simulink model "two_tanks_start"  (R2018a)
settings: Solver=ode45  StartTime=0.0  StopTime=250  RelTol=1e-3  EnableMultiTasking=on
PreLoadFcn:
  | rho = 1000;
  | A = 4;
  | g = 9.81;
  | R = 5;
  | W_in = 100;
  | h0 = 0;
  | hmax = 2;
settings Model: Creator=nicholas  LastModifiedBy=bneiswan
settings DataIOCC: LimitDataPoints=on  SaveFormat=Array  SignalLoggingName=sigsOut
settings OptimizationCC: BooleanDataType=off  OptimizeBlockIOStorage=off  BufferReuse=off  GlobalBufferReuse=off  ExpressionFolding=off  ExpressionDepthLimit=2147483647  LocalBlockOutputs=off  InitFltsAndDblsToZero=on  LifeSpan=inf  OptimizeDataStoreBuffers=off  BusAssignmentInplaceUpdate=off
settings DebuggingCC: SaveWithParameterizedLinksMsg=none  UnderspecifiedInitializationDetection=Classic  MergeDetectMultiDrivingBlocksExec=none  CheckExecutionContextPreStartOutputMsg=on  CheckExecutionContextRuntimeOutputMsg=on  SignalResolutionControl=TryResolveAllWithWarning  MultiTaskDSMMsg=warning  MultiTaskCondExecSysMsg=none  ParameterPrecisionLossMsg=none  FcnCallInpInsideContextMsg=warning  AllowSymbolicDim=off  StateNameClashWarn=warning  SFUnexpectedBacktrackingDiag=warning  SFNoUnconditionalDefaultTransitionDiag=warning  SFExecutionAtInitializationDiag=none
settings HardwareCC: ProdBitPerPointer=32  ProdBitPerSizeT=32  ProdBitPerPtrDiffT=32  ProdLargestAtomicFloat=None  ProdIntDivRoundTo=Undefined  ProdEndianess=Unspecified  ProdWordSize=32  ProdHWDeviceType=32-bit Generic  TargetUnknown=on
settings ModelReferenceCC: PropagateSignalLabelsOutOfModel=off
settings CodeAppCC: StateflowObjectComments=on
settings GRTTargetCC: TargetFcnLib=ansi_tfl_tmw.mat  TargetLangStandard=C89/C90 (ANSI)  GeneratePreprocessorConditionals=Disable all  CombineOutputUpdateFcns=off  GRTInterface=on
settings ConfigComp: CovMetricSettings=dw  CovHtmlReporting=on  CovSaveCumulativeToWorkspaceVar=on  CovSaveSingleToWorkspaceVar=on  CovExternalEMLEnable=off  CovSFcnEnable=off

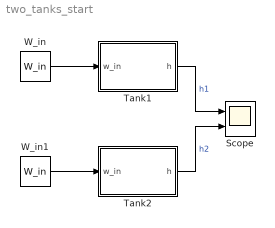
== system two_tanks_start ==
  Scope : Scope  NumInputPorts=2
  Tank1 : Subsystem
  Tank2 : Subsystem
  W_in : Constant  Value=W_in
  W_in1 : Constant  Value=W_in
  wires:
  Tank1/1(h) -> Scope/1  "h1"
  W_in/1 -> Tank1/1(w_in)
  W_in1/1 -> Tank2/1(w_in)
  Tank2/1(h) -> Scope/2  "h2"

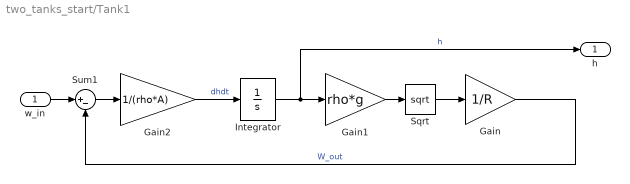
== system two_tanks_start/Tank1 ==
  w_in : Inport
  Gain : Gain  Gain=1/R  SaturateOnIntegerOverflow=on  OutDataTypeStr=Inherit: Same as input  ParamDataTypeStr=Inherit: Same as input
  Gain1 : Gain  Gain=rho*g  SaturateOnIntegerOverflow=on  OutDataTypeStr=Inherit: Same as input  ParamDataTypeStr=Inherit: Same as input
  Gain2 : Gain  Gain=1/(rho*A)  SaturateOnIntegerOverflow=on  OutDataTypeStr=Inherit: Same as input  ParamDataTypeStr=Inherit: Same as input
  Integrator : Integrator  InitialCondition=h0  UpperSaturationLimit=hmax  LowerSaturationLimit=0
      settings: AttributesFormatString=IC: %<InitialCondition>
  Sqrt : Sqrt  SaturateOnIntegerOverflow=on
  Sum1 : Sum  Inputs=|+-  SaturateOnIntegerOverflow=on  InputSameDT=on  OutDataTypeStr=Inherit: Same as first input
  h : Outport
  wires:
  Integrator/1 -> Gain1/1, h/1  "h"
  Gain1/1 -> Sqrt/1
  Sqrt/1 -> Gain/1
  Gain2/1 -> Integrator/1  "dhdt"
  Sum1/1 -> Gain2/1
  Gain/1 -> Sum1/2  "W_out"
  w_in/1 -> Sum1/1

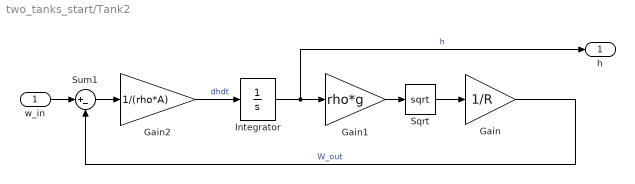
== system two_tanks_start/Tank2 ==
  w_in : Inport
  Gain : Gain  Gain=1/R  SaturateOnIntegerOverflow=on  OutDataTypeStr=Inherit: Same as input  ParamDataTypeStr=Inherit: Same as input
  Gain1 : Gain  Gain=rho*g  SaturateOnIntegerOverflow=on  OutDataTypeStr=Inherit: Same as input  ParamDataTypeStr=Inherit: Same as input
  Gain2 : Gain  Gain=1/(rho*A)  SaturateOnIntegerOverflow=on  OutDataTypeStr=Inherit: Same as input  ParamDataTypeStr=Inherit: Same as input
  Integrator : Integrator  InitialCondition=h0  UpperSaturationLimit=hmax  LowerSaturationLimit=0
      settings: AttributesFormatString=IC: %<InitialCondition>
  Sqrt : Sqrt  SaturateOnIntegerOverflow=on
  Sum1 : Sum  Inputs=|+-  SaturateOnIntegerOverflow=on  InputSameDT=on  OutDataTypeStr=Inherit: Same as first input
  h : Outport
  wires:
  w_in/1 -> Sum1/1
  Gain/1 -> Sum1/2  "W_out"
  Sum1/1 -> Gain2/1
  Gain2/1 -> Integrator/1  "dhdt"
  Sqrt/1 -> Gain/1
  Gain1/1 -> Sqrt/1
  Integrator/1 -> h/1, Gain1/1  "h"
